simulink model "SMC_TwoLink"  (R2020b)
settings: Solver=VariableStepAuto  StartTime=0.0  StopTime=20  RelTol=1e-3
libraries: checkpacklib x1
settings Model: OrderedModelArguments=off  Creator=MR.co  LastModifiedBy=Taha
settings DataIOCC: SaveFormat=Array  InspectSignalLogs=on

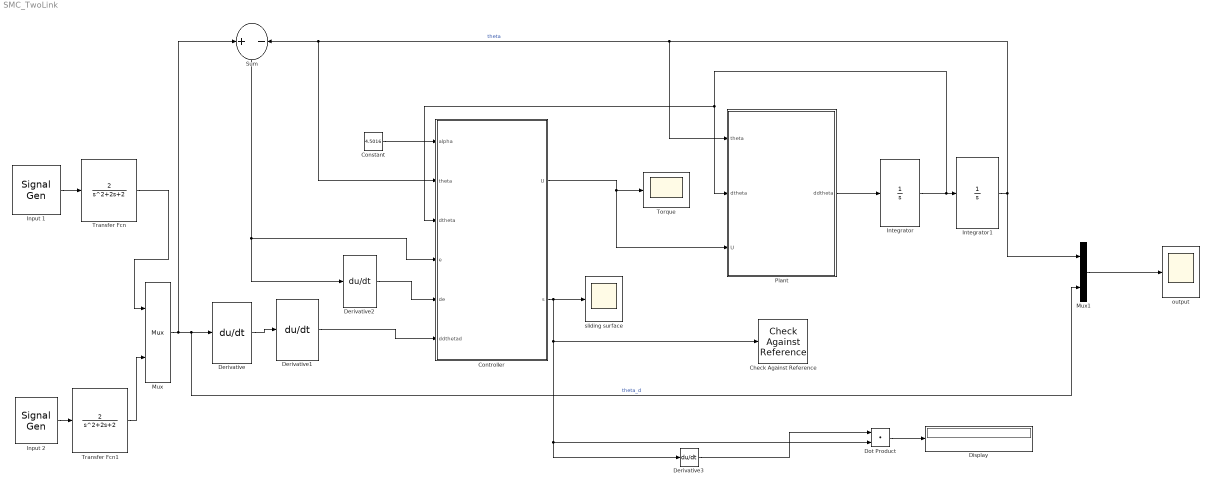
== system SMC_TwoLink ==
  Check Against Reference : checkpacklib/Check Against Reference  InstantiateOnLoad=on  enabled=on  stopWhenAssertionFail=off  export=off  ViewDlgPos=[]  OpenViewOnLoad=off  LaunchViewOnOpen=off  TimeUnits=seconds  EnableReferenceBound=on  AbsTolerance=eps^(1/3)  RelTolerance=0.01  ReferenceTimes=linspace(0,10)  ReferenceAmplitudes=1-exp(-linspace(0,10)/2)
      settings: SourceProductBaseCode=CT,ID,MT,SO
  Constant : Constant  Value=4.5016
  Controller : MATLAB Function  TreatAsAtomicUnit=on
  Derivative{,1..3} (4 alike) : Derivative
  Display : Display
  Dot Product : DotProduct  InputSameDT=on  OutDataTypeStr=Inherit: Inherit via internal rule
  Input 1 : SignalGenerator  Amplitude=2  Frequency=pi  Units=rad/sec
  Input 2 : SignalGenerator  WaveForm=square  Amplitude=3  Frequency=pi/2  Units=rad/sec
  Integrator : Integrator  InitialCondition=[0.5 0.5]
  Integrator1 : Integrator  InitialCondition=[0.5 0.5]
  Mux : Mux  Inputs=2
  Mux1 : Mux  Inputs=2
  Plant : MATLAB Function  TreatAsAtomicUnit=on
  Sum : Sum  Inputs=+|-
  Torque : Scope
  Transfer Fcn : TransferFcn  Numerator=[2]  Denominator=[1 2 2]
  Transfer Fcn1 : TransferFcn  Numerator=[2]  Denominator=[1 2 2]
  output : Scope
  sliding surface : Scope
  wires:
  Controller/1(U) -> Plant/3(U), Torque/1
  Plant/1(ddtheta) -> Integrator/1
  Integrator/1 -> Plant/2(dtheta), Controller/3(dtheta), Integrator1/1
  Input 1/1 -> Transfer Fcn/1
  Input 2/1 -> Transfer Fcn1/1
  Transfer Fcn1/1 -> Mux/2
  Transfer Fcn/1 -> Mux/1
  Derivative/1 -> Derivative1/1
  Derivative1/1 -> Controller/6(ddthetad)
  Integrator1/1 -> Mux1/1, Plant/1(theta), Controller/2(theta), Sum/2  "theta"
  Mux/1 -> Mux1/2, Derivative/1, Sum/1  "theta_d"
  Sum/1 -> Derivative2/1, Controller/4(e)
  Derivative2/1 -> Controller/5(de)
  Mux1/1 -> output/1
  Controller/2(s) -> Check Against Reference/1, Dot Product/2, Derivative3/1, sliding surface/1
  Dot Product/1 -> Display/1
  Derivative3/1 -> Dot Product/1
  Constant/1 -> Controller/1(alpha)

== matlab function SMC_TwoLink/Controller ==
  data: alpha input; theta input; U output; dtheta input; e input; de input; ddthetad input; s output
function [U , s]= fcn(alpha, theta , dtheta , e , de, ddthetad)


    L1 = 1; % m
    L2 = 1.2; % m
    
    Lc1 = .5; % m
    Lc2 = .6; % m
     
    m1 = 1; % Kg
    m2 = 2; % Kgkk
    
    I1 = 1/12 * m1 * L1^2;  %kg.N
    I2 = 1/12 * m2 * L2^2;  %kg.N

    g = 9.8; % m/s^2
   
    
    M11 = m1 * Lc1^2 + I1 + m2*(L1^2 + Lc2^2 + 2 * L1 * Lc2 * cos(theta(2))) + I2;
    M12 = m2 * L1 * Lc2 * cos(theta(2)) + m2 * Lc2^2 + I2;
    M22 = m2 * Lc2^2 + I2;
    M=[M11 M12;M12 M22];

    G1 = m1 * Lc1 * cos(theta(1)) + m2 * (Lc2 * cos(theta(1) + theta(2)) + L1 * cos(theta(1)));
    G2 = m2 * Lc2 * cos(theta(1) + theta(2));
    G=[G1*g;G2*g];
    
    F12 = m2 * L1 * Lc2 * sin(theta(2));
    C=[-F12*dtheta(2) -F12*(dtheta(1)+dtheta(2));F12*dtheta(1) 0];
  
    c = alpha* eye(2);
    ebs = beta * eye(2);
    
    
    s = de + c * e;
       
    s = de+ c*e + 5 * (e.^2);
    
   
    U = M * (ddthetad + c* de + ebs * sign(s)) + C * dtheta + G;
end

== matlab function SMC_TwoLink/Plant ==
  data: theta input; ddtheta output; dtheta input; U input
function ddtheta = fcn( theta , dtheta , U)


    L1 = 1; % m
    L2 = 1.2; % m
    
    Lc1 = .5; % m
    Lc2 = .6; % m
     
    m1 = 1; % Kg
    m2 = 2; % Kg
    
    I1 = 1/12 * m1 * L1^2;  %kg.N
    I2 = 1/12 * m2 * L2^2;  %kg.N

    g = 9.8; % m/s^2
   
    
    M11 = m1 * Lc1^2 + I1 + m2*(L1^2 + Lc2^2 + 2 * L1 * Lc2 * cos(theta(2))) + I2;
    M12 = m2 * L1 * Lc2 * cos(theta(2)) + m2 * Lc2^2 + I2;
    M22 = m2 * Lc2^2 + I2;
    M=[M11 M12;M12 M22];

    G1 = m1 * Lc1 * cos(theta(1)) + m2 * (Lc2 * cos(theta(1) + theta(2)) + L1 * cos(theta(1)));
    G2 = m2 * Lc2 * cos(theta(1) + theta(2));
    G=[G1*g;G2*g];
    
    F12 = m2 * L1 * Lc2 * sin(theta(2));
    C=[-F12*dtheta(2) -F12*(dtheta(1)+dtheta(2));F12*dtheta(1) 0];
    
    
    ddtheta = M\( U -C*dtheta -G );
